simulink model "pressurisation_system_model"  (R2025b)
settings: Solver=FixedStepAuto  StartTime=0.0  StopTime=1200.0  FixedStep=0.1  RelTol=1e-3
settings Model: PacingRate=10  Creator=domin  LastModifiedBy=domin

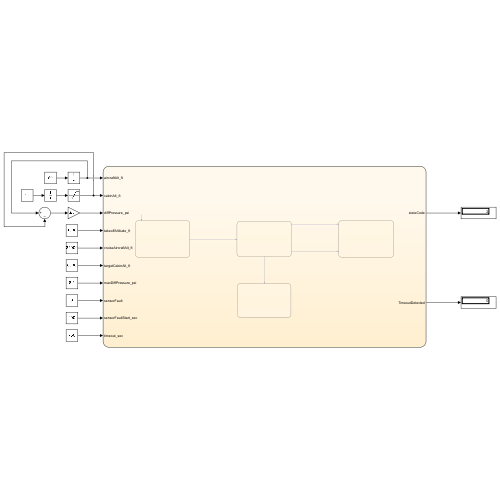
[thumbnail: Simulink's stored preview of the top-level diagram]
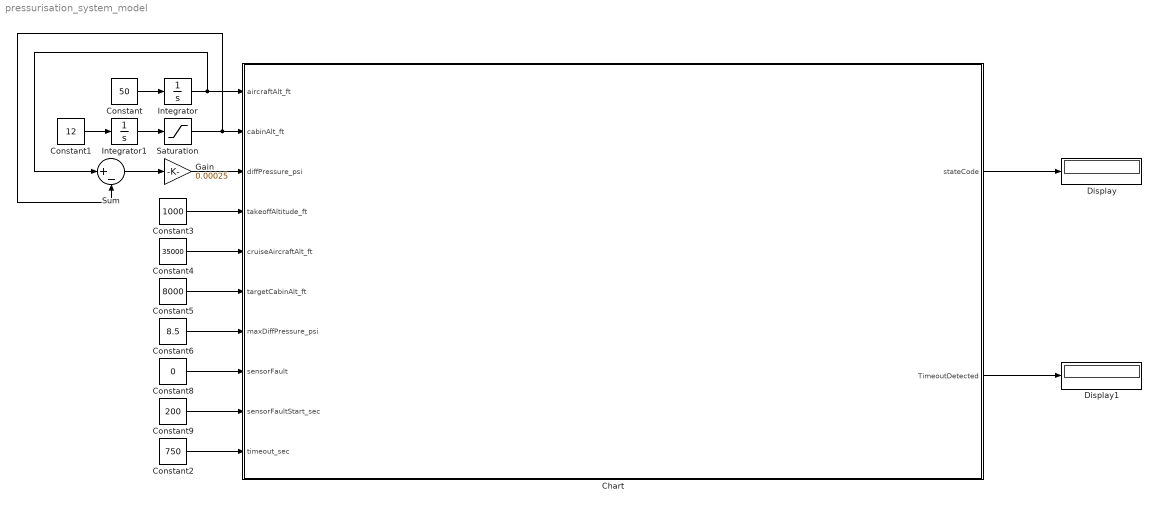
== system pressurisation_system_model ==
  Chart : Stateflow chart  TreatAsAtomicUnit=on
  Constant : Constant  Value=50
  Constant1 : Constant  Value=12
  Constant2 : Constant  Value=750
  Constant3 : Constant  Value=1000
  Constant4 : Constant  Value=35000
  Constant5 : Constant  Value=8000
  Constant6 : Constant  Value=8.5
  Constant8 : Constant  Value=0
  Constant9 : Constant  Value=200
  Display : Display
  Display1 : Display
  Gain : Gain  Gain=0.00025
  Integrator : Integrator
  Integrator1 : Integrator
  Saturation : Saturate  UpperLimit=8000  LowerLimit=0
  Sum : Sum  Inputs=|+-
  wires:
  Chart/1(stateCode) -> Display/1
  Gain/1 -> Chart/3(diffPressure_psi)
  Constant3/1 -> Chart/4(takeoffAltitude_ft)
  Constant4/1 -> Chart/5(cruiseAircraftAlt_ft)
  Constant5/1 -> Chart/6(targetCabinAlt_ft)
  Constant6/1 -> Chart/7(maxDiffPressure_psi)
  Constant8/1 -> Chart/8(sensorFault)
  Constant9/1 -> Chart/9(sensorFaultStart_sec)
  Constant/1 -> Integrator/1
  Integrator/1 -> Sum/1, Chart/1(aircraftAlt_ft)
  Constant1/1 -> Integrator1/1
  Sum/1 -> Gain/1
  Saturation/1 -> Chart/2(cabinAlt_ft), Sum/2
  Integrator1/1 -> Saturation/1
  Constant2/1 -> Chart/10(timeout_sec)
  Chart/2(TimeoutDetected) -> Display1/1

== stateflow chart pressurisation_system_model/Chart ==
  state GROUND
    entry:
    stateCode = 0;
  state FAULT
    entry:
    stateCode = 3;
  state PRESSURISING
    entry:
    stateCode = 1;
    TimeoutDetected = false;
    during:
    % REQ-05: set timeout flag if CRUISE
    % is not reached within the time threshold
    if after(timeout_sec, sec) && stateCode ~= 2
    TimeoutDetected = true;
    end
  state CRUISE
    entry:
    stateCode = 2;
  (default) -> GROUND
  PRESSURISING -> FAULT [order 2] : % REQ-04: detect and flag sensor fault condition
      | % REQ-06: transition to FAULT following sensor fault detection
      | [sensorFault && t >= sensorFaultStart_sec]
  GROUND -> PRESSURISING : % Aircraft takeoff detected: begin pressurisation sequence
      | % Precondition for meeting REQ-01 under nominal operation
      | [aircraftAlt_ft >= takeoffAltitude_ft]
  PRESSURISING -> FAULT [order 3] : % REQ-03: pressure safety limit exceeded
      | % transition to FAULT to prevent unsafe operation
      | [diffPressure_psi > maxDiffPressure_psi]
  PRESSURISING -> CRUISE [order 1] : % REQ-01/REQ-02: enter CRUISE when aircraft reaches cruise altitude
      | % and cabin altitude is within acceptable tolerance of target value
      | [aircraftAlt_ft >= cruiseAircraftAlt_ft && abs(cabinAlt_ft - targetCabinAlt_ft) <= 100]
  data: aircraftAlt_ft input; cabinAlt_ft input; diffPressure_psi input; takeoffAltitude_ft input; cruiseAircraftAlt_ft input; targetCabinAlt_ft input; maxDiffPressure_psi input; sensorFault input; sensorFaultStart_sec input; timeout_sec input double; stateCode output; TimeoutDetected output boolean =false
